simulink library "resettableTimer_ul"  (R2018a)
settings: Solver=VariableStepAuto  StartTime=0.0  StopTime=10.0  RelTol=1e-3
libraries: dspsigops x1
settings Model: Creator=mcobb  LastModifiedBy=mcobb

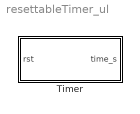
== system resettableTimer_ul ==
  Timer : Subsystem

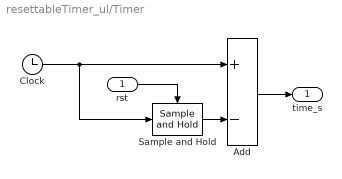
== system resettableTimer_ul/Timer ==
  rst : Inport
  Add : Sum  Inputs=+-
  Clock : Clock
  Sample and Hold : dspsigops/Sample and Hold  trig=Rising edge  initCond=0  latchinput=off
  time_s : Outport
  wires:
  Clock/1 -> Sample and Hold/1, Add/1
  rst/1 -> Sample and Hold/Trigger
  Sample and Hold/1 -> Add/2
  Add/1 -> time_s/1
